simulink model "part2_cnt12"  (R2016b)
settings: Solver=VariableStepAuto  StartTime=0.0  StopTime=10.0  RelTol=1e-3
values from neighbouring files (symbols this model uses):
  Acl = A - B*k    [sara.m]
  B = [0;0.2263;0;-0.3565]    [4_5864020115967706803.m]    (also in NYQ.m; Nq_cntrl.m; Nquist.m; main.m)
  k = 1    [4_5864020115967706803.m]    (also in main.m = place(A,B,P); part_2.m; sara.m = place(A,B,P))
  Kf = 1/Kdc    [sara.m]
undefined symbols (not defined in the file or in its folder): a1, a2, b1, b2
settings Model: Creator=ASUS  LastModifiedBy=ASUS

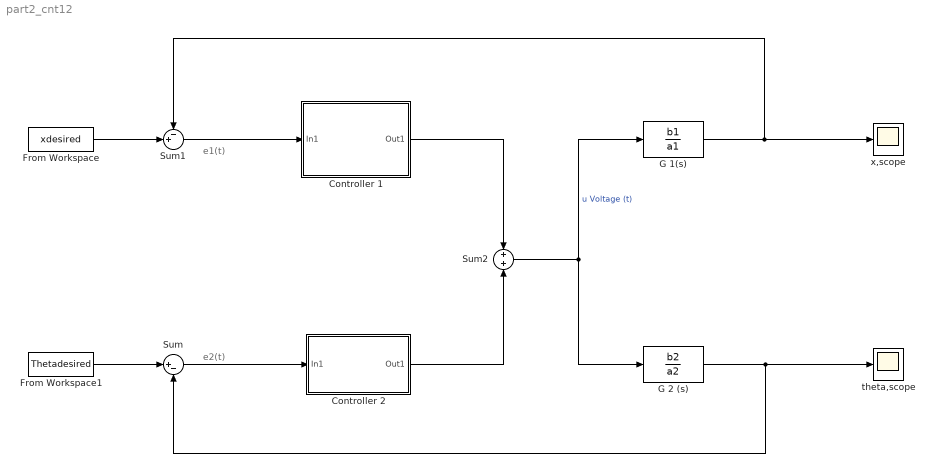
== system part2_cnt12 ==
  note: e2(t)
  note: e1(t)
  "Controller 1 " : Subsystem
  Controller 2 : Subsystem
  From Workspace : FromWorkspace  VariableName=xdesired  SampleTime=0
  From Workspace1 : FromWorkspace  VariableName=Thetadesired  SampleTime=0
  G 1(s) : TransferFcn  Numerator=b1  Denominator=a1
  G 2 (s) : TransferFcn  Numerator=b2  Denominator=a2
  Sum : Sum  Inputs=|+-
  Sum1 : Sum  Inputs=-+|
  Sum2 : Sum  Inputs=+|+
  theta,scope : Scope
  x,scope : Scope
  wires:
  Sum1/1 -> "Controller 1 "/1(In1)
  "Controller 1 "/1(Out1) -> Sum2/1
  Sum/1 -> Controller 2/1(In1)
  Controller 2/1(Out1) -> Sum2/2
  Sum2/1 -> G 2 (s)/1, G 1(s)/1  "u Voltage (t)"
  G 1(s)/1 -> x,scope/1, Sum1/1
  G 2 (s)/1 -> theta,scope/1, Sum/2
  From Workspace/1 -> Sum1/2
  From Workspace1/1 -> Sum/1

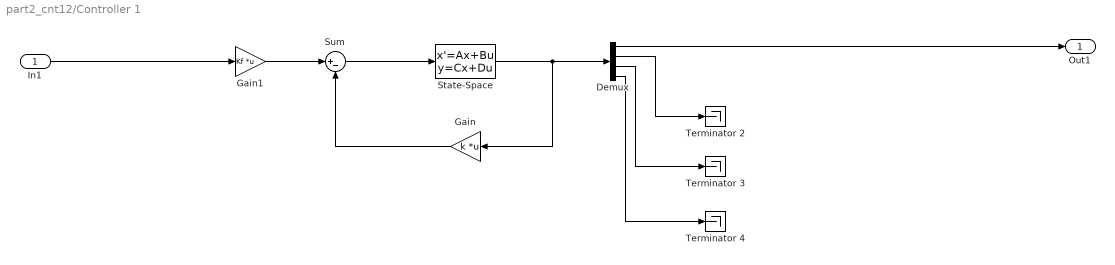
== system part2_cnt12/Controller 1  ==
  In1 : Inport
  Demux : Demux
  Gain : Gain  Gain=k  Multiplication=Matrix(K*u)
  Gain1 : Gain  Gain=Kf  Multiplication=Matrix(K*u)
  State-Space : StateSpace  A=Acl  B=B  C=eye(4)  D=[0;0;0;0]  X0=0
  Sum : Sum  Inputs=|+-
  Terminator 2 : Terminator
  Terminator 3 : Terminator
  "Terminator 4 " : Terminator
  Out1 : Outport
  wires:
  Gain/1 -> Sum/2
  State-Space/1 -> Gain/1, Demux/1
  Sum/1 -> State-Space/1
  Demux/4 -> "Terminator 4 "/1
  In1/1 -> Gain1/1
  Gain1/1 -> Sum/1
  Demux/2 -> Terminator 2/1
  Demux/3 -> Terminator 3/1
  Demux/1 -> Out1/1

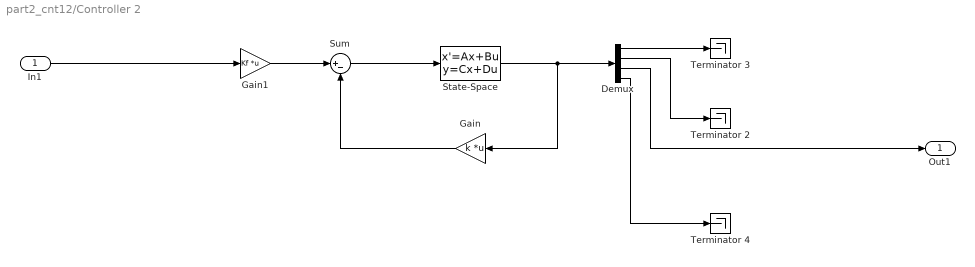
== system part2_cnt12/Controller 2 ==
  In1 : Inport
  Demux : Demux
  Gain : Gain  Gain=k  Multiplication=Matrix(K*u)
  Gain1 : Gain  Gain=Kf  Multiplication=Matrix(K*u)
  State-Space : StateSpace  A=Acl  B=B  C=eye(4)  D=[0;0;0;0]  X0=0
  Sum : Sum  Inputs=|+-
  Terminator 2 : Terminator
  Terminator 3 : Terminator
  "Terminator 4 " : Terminator
  Out1 : Outport
  wires:
  Demux/1 -> Terminator 3/1
  Demux/2 -> Terminator 2/1
  Demux/4 -> "Terminator 4 "/1
  In1/1 -> Gain1/1
  State-Space/1 -> Gain/1, Demux/1
  Gain1/1 -> Sum/1
  Gain/1 -> Sum/2
  Sum/1 -> State-Space/1
  Demux/3 -> Out1/1
